simulink model "Subsystem"  (R2020b)
settings: Solver=FixedStepAuto  StartTime=0.0  StopTime=10.0  FixedStep=1  MaxStep=0.01  RelTol=1e-3
settings Model: Creator=lalit  LastModifiedBy=lalit
settings DataIOCC: SaveOutput=off  SaveTime=off

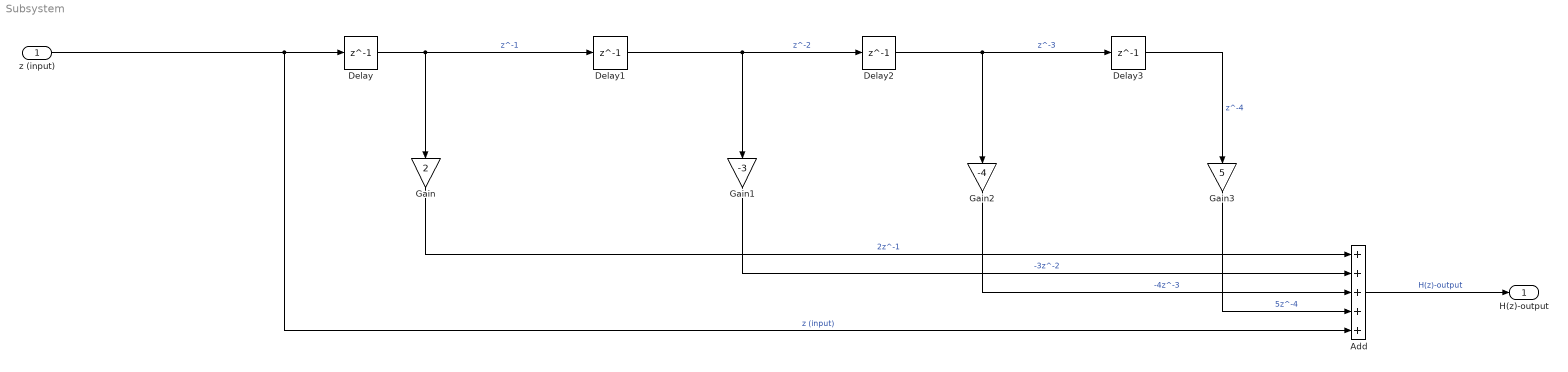
== system Subsystem ==
  z (input) : Inport  OutDataTypeStr=double  PortDimensions=[1 1]  SampleTime=[1,0]
  Add : Sum  Inputs=+++++
  Delay{,1..3} (4 alike) : Delay  DelayLength=1
  Gain : Gain  Gain=2
  Gain1 : Gain  Gain=-3
  Gain2 : Gain  Gain=-4
  Gain3 : Gain  Gain=5
  H(z)-output : Outport  OutDataTypeStr=double  PortDimensions=[1 1]  SampleTime=[1,0]
  wires:
  Gain1/1 -> Add/2  "-3z^-2"
  z (input)/1 -> Delay/1, Add/5  "z (input)"
  Add/1 -> H(z)-output/1  "H(z)-output"
  Delay3/1 -> Gain3/1  "z^-4"
  Delay2/1 -> Delay3/1, Gain2/1  "z^-3"
  Delay/1 -> Gain/1, Delay1/1  "z^-1"
  Gain3/1 -> Add/4  "5z^-4"
  Gain2/1 -> Add/3  "-4z^-3"
  Delay1/1 -> Delay2/1, Gain1/1  "z^-2"
  Gain/1 -> Add/1  "2z^-1"
